simulink model "rcrc_cntrl_sim"  (R2024a)
settings: Solver=ode23tb  StartTime=0.0  StopTime=0.1  RelTol=1e-3
values from neighbouring files (symbols this model uses):
  A = [-(R1+R2)/(R1*R2*C1),  1/(R2*C1) ... (first row only)    [rcrc_ini.m]
  B = [1/(R1*C1) ... (first row only)    [rcrc_ini.m]
  C = [0 1]    [rcrc_ini.m]
  C1 = 470e-9    (= 4.7e-07)    [rcrc_ini.m]
  C2 = C1    (= 4.7e-07)    [rcrc_ini.m]
  H = place(A.', C.', 3 * [-500 + 500*1i; -500 - 500*1i])'    [rcrc_ini.m]
  K = place(A, B, 2 * [-500 + 500*1i; -500 - 500*1i])    [rcrc_ini.m]
  R1 = 4.7e3    (= 4700)    [rcrc_ini.m]
  R2 = R1    (= 4700)    [rcrc_ini.m]
  V = -1 / (C * (A - B*K)^-1 * B)    [rcrc_ini.m]
libraries: cstblocks x1
settings Model: Creator=pmic  LastModifiedBy=pichim
settings SolverCC: AlgebraicLoopSolver=TrustRegion
settings DebuggingCC: UnconnectedInputMsg=warning  UnconnectedOutputMsg=warning  UnconnectedLineMsg=warning
settings ModelReferenceCC: EnableRefExpFcnMdlSchedulingChecks=on
settings RTWCC: GPUComputeCapability=3.5  DLArmComputeVersion=19.05

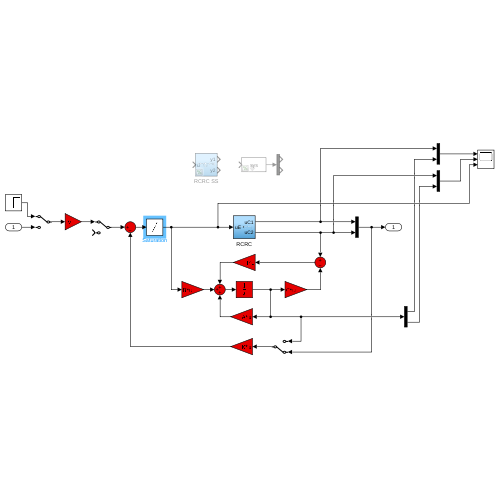
[thumbnail: Simulink's stored preview of the top-level diagram]
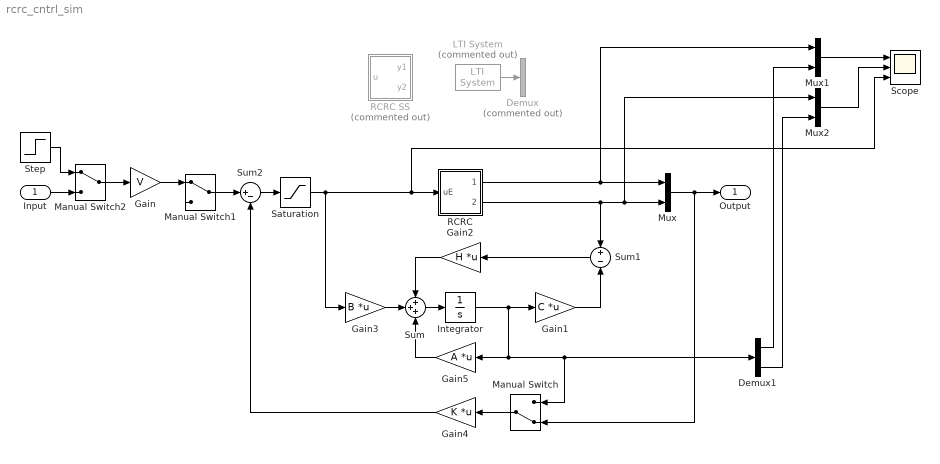
== system rcrc_cntrl_sim ==
  Input : Inport
  Demux : Demux  Commented=on  Outputs=2
  Demux1 : Demux  Outputs=2
  Gain : Gain  Gain=V
  Gain1 : Gain  Gain=C  Multiplication=Matrix(K*u)
  Gain2 : Gain  Gain=H  Multiplication=Matrix(K*u)
  Gain3 : Gain  Gain=B  Multiplication=Matrix(K*u)
  Gain4 : Gain  Gain=K  Multiplication=Matrix(K*u)
  Gain5 : Gain  Gain=A  Multiplication=Matrix(K*u)
  Integrator : Integrator
  LTI System : cstblocks/LTI System  Commented=on  sys=sys  IC=[]  PadeOrder=0
  Manual Switch : ManualSwitch  CurrentSetting=0
  Manual Switch1 : ManualSwitch
  Manual Switch2 : ManualSwitch
  Mux : Mux  Inputs=2
  Mux1 : Mux  Inputs=2
  Mux2 : Mux  Inputs=2
  RCRC : Subsystem
  RCRC SS : Subsystem  Commented=on
  Saturation : Saturate  UpperLimit=3.3/2  LowerLimit=-3.3/2
  Scope : Scope  NumInputPorts=3
  Step : Step  Time=0.05  After=0.5  SampleTime=0
  Sum : Sum  Inputs=+++
  Sum1 : Sum  Inputs=+|-
  Sum2 : Sum  Inputs=|+-
  Output : Outport
  wires:
  Sum/1 -> Integrator/1
  Gain5/1 -> Sum/3
  Integrator/1 -> Gain1/1, Demux1/1, Manual Switch/1, Gain5/1
  Gain3/1 -> Sum/2
  Gain1/1 -> Sum1/2
  Gain2/1 -> Sum/1
  Sum1/1 -> Gain2/1
  RCRC/1(uC1) -> Mux1/1, Mux/1
  RCRC/2(uC2) -> Sum1/1, Mux2/1, Mux/2
  Manual Switch/1 -> Gain4/1
  Mux/1 -> Output/1, Manual Switch/2
  Sum2/1 -> Saturation/1
  Gain4/1 -> Sum2/2
  Manual Switch1/1 -> Sum2/1
  Gain/1 -> Manual Switch1/1
  LTI System/1 -> Demux/1
  Manual Switch2/1 -> Gain/1
  Input/1 -> Manual Switch2/2
  Step/1 -> Manual Switch2/1
  Saturation/1 -> Gain3/1, Scope/3, RCRC/1(uE)
  Demux1/1 -> Mux1/2
  Demux1/2 -> Mux2/2
  Mux2/1 -> Scope/2
  Mux1/1 -> Scope/1

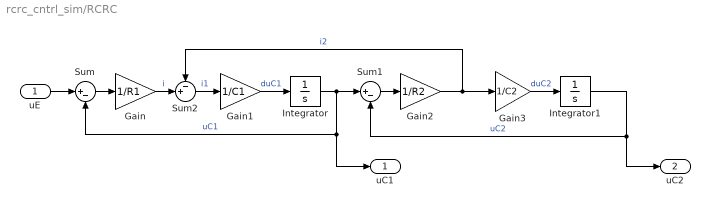
== system rcrc_cntrl_sim/RCRC ==
  uE : Inport
  Gain : Gain  Gain=1/R1
  Gain1 : Gain  Gain=1/C1
  Gain2 : Gain  Gain=1/R2
  Gain3 : Gain  Gain=1/C2
  Integrator : Integrator
  Integrator1 : Integrator
  Sum : Sum  Inputs=|+-
  Sum1 : Sum  Inputs=|+-
  Sum2 : Sum  Inputs=-+|
  uC1 : Outport
  uC2 : Outport  Port=2
  wires:
  Sum2/1 -> Gain1/1  "i1"
  Gain3/1 -> Integrator1/1  "duC2"
  uE/1 -> Sum/1
  Sum/1 -> Gain/1
  Gain/1 -> Sum2/2  "i"
  Gain1/1 -> Integrator/1  "duC1"
  Sum1/1 -> Gain2/1
  Gain2/1 -> Gain3/1, Sum2/1  "i2"
  Integrator1/1 -> uC2/1, Sum1/2  "uC2"
  Integrator/1 -> uC1/1, Sum/2, Sum1/1  "uC1"

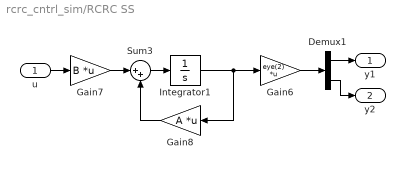
== system rcrc_cntrl_sim/RCRC SS ==
  u : Inport
  Demux1 : Demux  Outputs=2
  Gain6 : Gain  Gain=eye(2)  Multiplication=Matrix(K*u)
  Gain7 : Gain  Gain=B  Multiplication=Matrix(K*u)
  Gain8 : Gain  Gain=A  Multiplication=Matrix(K*u)
  Integrator1 : Integrator
  Sum3 : Sum  Inputs=|++
  y1 : Outport
  y2 : Outport  Port=2
  wires:
  Gain8/1 -> Sum3/2
  Gain7/1 -> Sum3/1
  Sum3/1 -> Integrator1/1
  Integrator1/1 -> Gain6/1, Gain8/1
  Demux1/2 -> y2/1
  Gain6/1 -> Demux1/1
  Demux1/1 -> y1/1
  u/1 -> Gain7/1
